simulink model "ass6_4"  (R2023a)
settings: Solver=VariableStepAuto  StartTime=0.0  StopTime=10.0  RelTol=1e-3
settings Model: Creator=Taniya Baral  LastModifiedBy=Taniya Baral

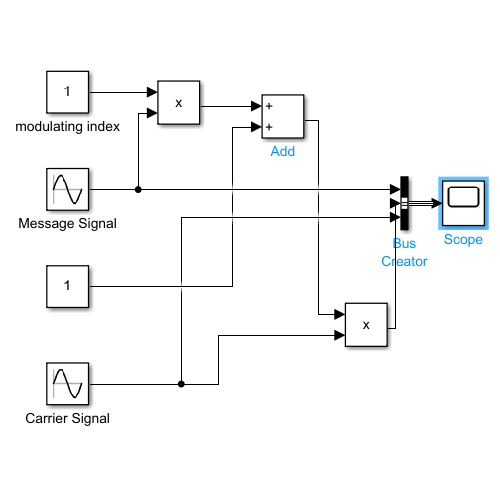
[thumbnail: Simulink's stored preview of the top-level diagram]
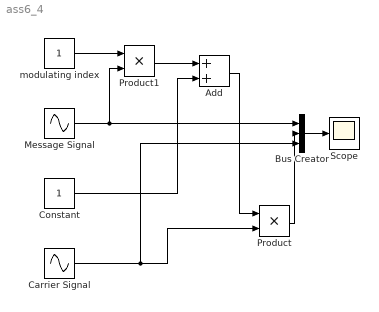
== system ass6_4 ==
  Add : Sum
  Bus Creator : BusCreator  Inputs=3
  Carrier Signal : Sin  Frequency=2*pi  Phase=180  SampleTime=0
  Constant : Constant
  Message Signal : Sin  Frequency=2*pi  Phase=180  SampleTime=0
  Product : Product
  Product1 : Product
  Scope : Scope
  modulating index : Constant
  wires:
  modulating index/1 -> Product1/1
  Message Signal/1 -> Bus Creator/1, Product1/2
  Constant/1 -> Add/2
  Product1/1 -> Add/1
  Add/1 -> Product/1
  Carrier Signal/1 -> Bus Creator/3, Product/2
  Product/1 -> Bus Creator/2
  Bus Creator/1 -> Scope/1
